simulink model "lab3Synth"  (Simulink 8.6)
settings: Solver=ode45  SolverMode=SingleTasking  StartTime=0.0  StopTime=50  MaxStep=0.005  RelTol=1e-3  AbsTol=1e-6
settings Model: Creator=vise  LastModifiedBy=EmanTnuocca  ExtModeTrigMode=oneshot  ExtModeArmWhenConnect=off
settings DataIOCC: LimitDataPoints=off
settings OptimizationCC: BlockReduction=off  BooleanDataType=off  ExpressionDepthLimit=128
settings DebuggingCC: SaveWithParameterizedLinksMsg=none  SignalResolutionControl=TryResolveAllWithWarning  SolverPrmCheckMsg=none  MultiTaskDSMMsg=warning  MultiTaskCondExecSysMsg=none  FcnCallInpInsideContextMsg=EnableAllAsError  StateNameClashWarn=none
settings HardwareCC: ProdBitPerPointer=64  ProdLargestAtomicFloat=Float  ProdIntDivRoundTo=Zero  ProdEndianess=LittleEndian  ProdWordSize=64  ProdHWDeviceType=Intel->x86-64 (Windows64)  TargetUnknown=on
settings RTWCC: TemplateMakefile=grt_unix.tmf
settings GRTTargetCC: GeneratePreprocessorConditionals=Use local settings
settings ConfigComp: CovModelRefEnable=off

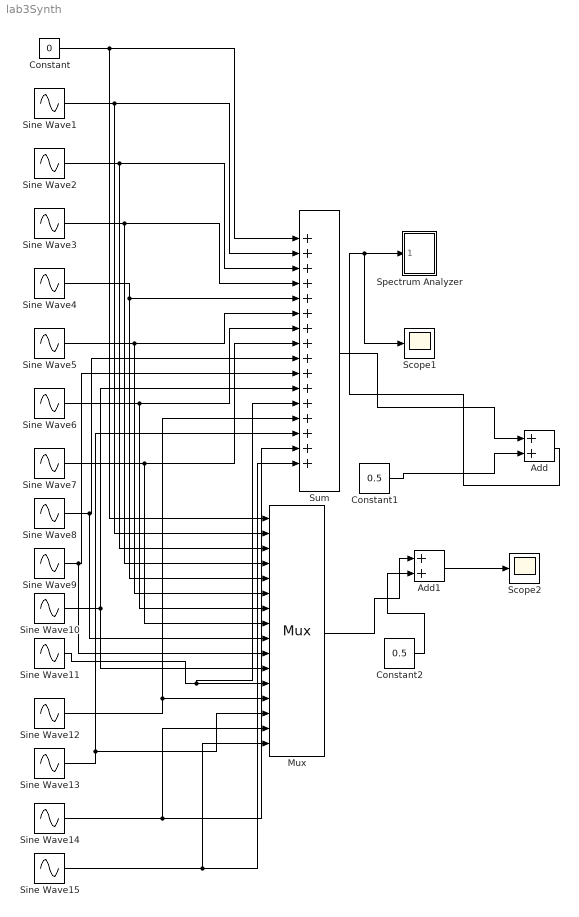
== system lab3Synth ==
  Add : Sum
  Add1 : Sum
  Constant : Constant  Value=0
  Constant1 : Constant  Value=0.5
  Constant2 : Constant  Value=0.5
  Mux : Mux  Inputs=16
  Scope1 : Scope
  Scope2 : Scope
  Sine Wave1 : Sin  Amplitude=4/pi  Frequency=2*pi  SampleTime=0
  Sine Wave10 : Sin  Amplitude=4/(19*pi)  Frequency=19*2*pi  SampleTime=0
  Sine Wave11 : Sin  Amplitude=4/(21*pi)  Frequency=21*2*pi  SampleTime=0
  Sine Wave12 : Sin  Amplitude=4/(23*pi)  Frequency=23*2*pi  SampleTime=0
  Sine Wave13 : Sin  Amplitude=4/(25*pi)  Frequency=25*2*pi  SampleTime=0
  Sine Wave14 : Sin  Amplitude=4/(27*pi)  Frequency=27*2*pi  SampleTime=0
  Sine Wave15 : Sin  Amplitude=4/(29*pi)  Frequency=29*2*pi  SampleTime=0
  Sine Wave2 : Sin  Amplitude=4/(3*pi)  Frequency=3*2*pi  SampleTime=0
  Sine Wave3 : Sin  Amplitude=4/(5*pi)  Frequency=5*2*pi  SampleTime=0
  Sine Wave4 : Sin  Amplitude=4/(7*pi)  Frequency=7*2*pi  SampleTime=0
  Sine Wave5 : Sin  Amplitude=4/(9*pi)  Frequency=9*2*pi  SampleTime=0
  Sine Wave6 : Sin  Amplitude=4/(11*pi)  Frequency=11*2*pi  SampleTime=0
  Sine Wave7 : Sin  Amplitude=4/(13*pi)  Frequency=13*2*pi  SampleTime=0
  Sine Wave8 : Sin  Amplitude=4/(15*pi)  Frequency=15*2*pi  SampleTime=0
  Sine Wave9 : Sin  Amplitude=4/(17*pi)  Frequency=17*2*pi  SampleTime=0
  Spectrum Analyzer : Subsystem  mask(Spectrum analyzer.){N=1024, T_s=0.01, plot_period=10}
      mask prompts: N "Number of sample points:"; T_s "Sampling period (sec):"; plot_period "Plotting Period (sec):"
      mask Help: EE438 Lab utility; See Prof. Bouman.
      mask Display: plot(0,0,100,100,[14,91,91,14,14],[86,86,40,40,86],[85,82,80,79,75,67,63,60,57,53,41,36,33,27,24],[49,50,53,50,49,51,54,66,54,50,50,52,81,51,49])
  Sum : Sum  Inputs=++++++++++++++++  SaturateOnIntegerOverflow=on  InputSameDT=on  OutDataTypeStr=Inherit: Same as first input
  wires:
  Add/1 -> Scope1/1, Spectrum Analyzer/1(input signal)
  Sine Wave7/1 -> Mux/8, Sum/8
  Sine Wave6/1 -> Mux/7, Sum/7
  Sine Wave5/1 -> Mux/6, Sum/6
  Sine Wave4/1 -> Mux/5, Sum/5
  Sine Wave3/1 -> Mux/4, Sum/4
  Sine Wave2/1 -> Mux/3, Sum/3
  Sine Wave1/1 -> Mux/2, Sum/2
  Constant/1 -> Mux/1, Sum/1
  Sine Wave8/1 -> Mux/9, Sum/9
  Sine Wave9/1 -> Mux/10, Sum/10
  Sine Wave10/1 -> Sum/11, Mux/11
  Sine Wave11/1 -> Sum/12, Mux/12
  Sine Wave12/1 -> Sum/13, Mux/13
  Sine Wave13/1 -> Sum/14, Mux/14
  Sine Wave14/1 -> Mux/15, Sum/15
  Sine Wave15/1 -> Mux/16, Sum/16
  Constant1/1 -> Add/2
  Sum/1 -> Add/1
  Constant2/1 -> Add1/2
  Mux/1 -> Add1/1
  Add1/1 -> Scope2/1

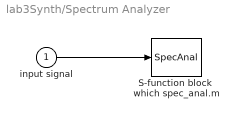
== system lab3Synth/Spectrum Analyzer ==
  input signal : Inport
  S-function block  which spec_anal.m : S-Function  FunctionName=SpecAnal  Parameters=N,T_s,plot_period  SFunctionDeploymentMode=off  EnableBusSupport=off
  wires:
  input signal/1 -> S-function block  which spec_anal.m/1
